simulink model "simulation"  (R2022b)
settings: Solver=VariableStepAuto  StartTime=0.0  StopTime=80000.0  FixedStep=0.1  MinStep=0.1  RelTol=1e-3
settings Model: Creator=umber  LastModifiedBy=umber
settings DataIOCC: ReturnWorkspaceOutputs=off

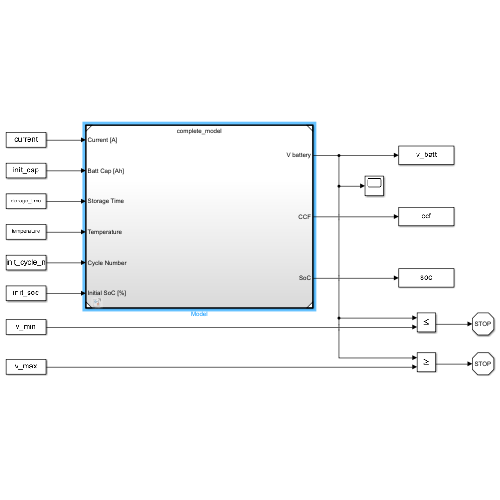
[thumbnail: Simulink's stored preview of the top-level diagram]
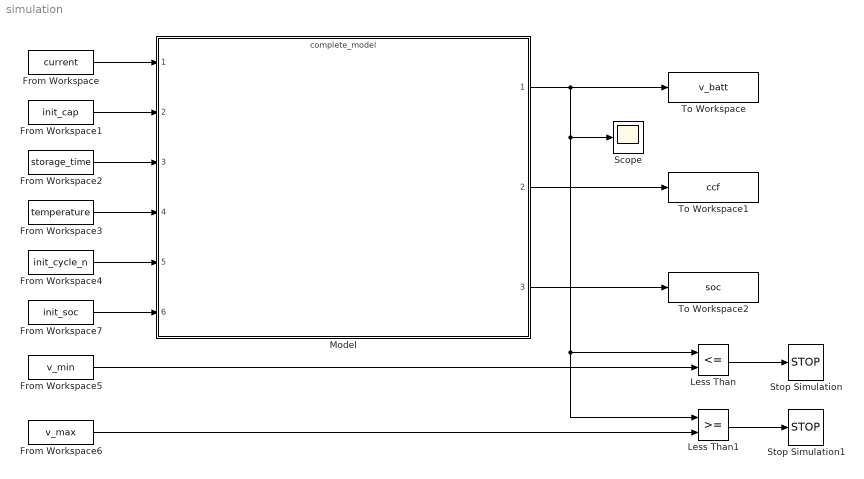
== system simulation ==
  From Workspace : FromWorkspace  VariableName=current
  From Workspace1 : FromWorkspace  VariableName=init_cap
  From Workspace2 : FromWorkspace  VariableName=storage_time
  From Workspace3 : FromWorkspace  VariableName=temperature
  From Workspace4 : FromWorkspace  VariableName=init_cycle_n
  From Workspace5 : FromWorkspace  VariableName=v_min  OutputAfterFinalValue=Holding final value
  From Workspace6 : FromWorkspace  VariableName=v_max  OutputAfterFinalValue=Holding final value
  From Workspace7 : FromWorkspace  VariableName=init_soc
  Less Than : RelationalOperator  Operator=<=  OutDataTypeStr=boolean  RndMeth=Simplest  InputSameDT=off
  Less Than1 : RelationalOperator  OutDataTypeStr=boolean  RndMeth=Simplest  InputSameDT=off
  Model : ModelReference  ModelNameDialog=complete_model.slx  SimulationMode=Normal  ModelReferenceVersion=2.37
  Scope : Scope
  Stop Simulation : Stop
  Stop Simulation1 : Stop
  To Workspace : ToWorkspace  VariableName=v_batt  SaveFormat=Timeseries  SampleTime=-1
      settings: Save2DSignal=2-D array (concatenate along first dimension)
  To Workspace1 : ToWorkspace  VariableName=ccf  SaveFormat=Timeseries  SampleTime=-1
      settings: Save2DSignal=2-D array (concatenate along first dimension)
  To Workspace2 : ToWorkspace  VariableName=soc  SaveFormat=Timeseries  SampleTime=-1
      settings: Save2DSignal=2-D array (concatenate along first dimension)
  wires:
  From Workspace/1 -> Model/1
  From Workspace1/1 -> Model/2
  From Workspace4/1 -> Model/5
  From Workspace3/1 -> Model/4
  From Workspace2/1 -> Model/3
  Model/1 -> Less Than1/1, Less Than/1, Scope/1, To Workspace/1
  From Workspace5/1 -> Less Than/2
  Model/2 -> To Workspace1/1
  From Workspace6/1 -> Less Than1/2
  Less Than1/1 -> Stop Simulation1/1
  From Workspace7/1 -> Model/6
  Less Than/1 -> Stop Simulation/1
  Model/3 -> To Workspace2/1
